simulink model "nonlin_model"  (Simulink 7.3)
settings: Solver=ode113  SolverMode=SingleTasking  StartTime=0  StopTime=0.02  RelTol=1e-3  AbsTol=1e-3
libraries: simulink x3
settings Model: Creator=gladkikh  LastModifiedBy=cubesun  BufferReuse=off
settings SolverCC: ZeroCrossAlgorithm=Adaptive
settings DataIOCC: LimitDataPoints=off  SignalLoggingName=sigsOut
settings OptimizationCC: BlockReduction=off  BooleanDataType=off  InlineParams=on  BufferReuse=off  InitFltsAndDblsToZero=on
settings DebuggingCC: AlgebraicLoopMsg=none  SaveWithParameterizedLinksMsg=none  SignalResolutionControl=TryResolveAllWithWarning  SolverPrmCheckMsg=none  MultiTaskDSMMsg=warning  MultiTaskCondExecSysMsg=none  UnconnectedInputMsg=none  UnconnectedOutputMsg=none  UnconnectedLineMsg=none  StrictBusMsg=None
settings HardwareCC: TargetEndianess=LittleEndian  TargetHWDeviceType=MATLAB Host  ProdEqTarget=off
settings RTWCC: IncludeERTFirstTime=on
settings GRTTargetCC: TargetFcnLib=ansi_tfl_tmw.mat

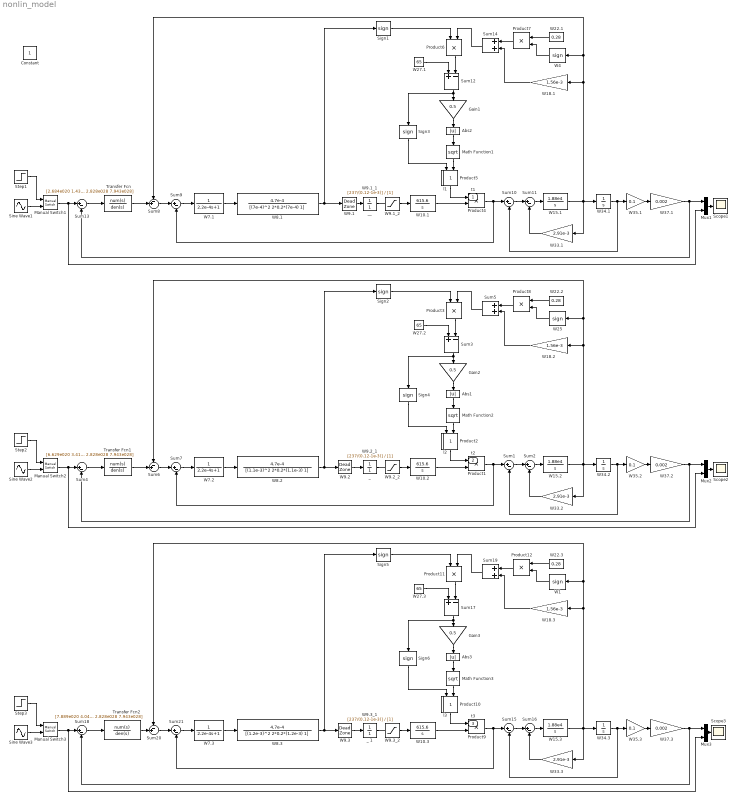
== system nonlin_model ==
  " W9.1_1" : TransferFcn  Numerator=[237/(0.12-1e-3)]  Denominator=[1]
  " W9.2_1" : TransferFcn  Numerator=[237/(0.12-1e-3)]  Denominator=[1]
  " W9.3_1" : TransferFcn  Numerator=[237/(0.12-1e-3)]  Denominator=[1]
  Abs1 : Abs  SaturateOnIntegerOverflow=on
  Abs2 : Abs  SaturateOnIntegerOverflow=on
  Abs3 : Abs  SaturateOnIntegerOverflow=on
  Gain1 : Gain  Gain=0.5  ParameterDataType=sfix(16)  ParameterScaling=2^0  OutDataType=sfix(16)  OutScaling=2^0  SaturateOnIntegerOverflow=on  OutDataTypeStr=Inherit: Same as input  ParamDataTypeStr=Inherit: Same as input
  Gain2 : Gain  Gain=0.5  ParameterDataType=sfix(16)  ParameterScaling=2^0  OutDataType=sfix(16)  OutScaling=2^0  SaturateOnIntegerOverflow=on  OutDataTypeStr=Inherit: Same as input  ParamDataTypeStr=Inherit: Same as input
  Gain3 : Gain  Gain=0.5  ParameterDataType=sfix(16)  ParameterScaling=2^0  OutDataType=sfix(16)  OutScaling=2^0  SaturateOnIntegerOverflow=on  OutDataTypeStr=Inherit: Same as input  ParamDataTypeStr=Inherit: Same as input
  Manual Switch1 : simulink/Signal Routing/Manual Switch  SystemSampleTime=-1  sw=1  action=0  varsize=off
  Manual Switch2 : simulink/Signal Routing/Manual Switch  SystemSampleTime=-1  sw=0  action=0  varsize=off
  Manual Switch3 : simulink/Signal Routing/Manual Switch  SystemSampleTime=-1  sw=0  action=0  varsize=off
  Math Function1 : Math  Operator=sqrt  OutDataType=sfix(16)  OutScaling=2^0  SaturateOnIntegerOverflow=on
  Math Function2 : Math  Operator=sqrt  OutDataType=sfix(16)  OutScaling=2^0  SaturateOnIntegerOverflow=on
  Math Function3 : Math  Operator=sqrt  OutDataType=sfix(16)  OutScaling=2^0  SaturateOnIntegerOverflow=on
  Mux1 : Mux  Inputs=2
  Mux2 : Mux  Inputs=2
  Mux3 : Mux  Inputs=2
  Product{1..12} (12 alike) : Product  OutDataType=sfix(16)  OutScaling=2^0  SaturateOnIntegerOverflow=on  InputSameDT=on  OutDataTypeStr=Inherit: Same as first input
  Scope1 : Scope
      settings: TimeRange=0.01  YMin=0.985  YMax=1.035
  Scope2 : Scope
      settings: YMin=-1  YMax=1
  Scope3 : Scope
      settings: YMin=-1  YMax=1  SaveName=ScopeData2
  Sign{1..6} (6 alike) : Signum
  Sine Wave1 : Sin  Amplitude=1  Bias=0  Frequency=3100  Phase=0  Samples=10  SampleTime=0  Offset=0
  Sine Wave2 : Sin  Amplitude=1  Bias=0  Frequency=3100  Phase=0  Samples=10  SampleTime=0  Offset=0
  Sine Wave3 : Sin  Amplitude=1  Bias=0  Frequency=3100  Phase=0  Samples=10  SampleTime=0  Offset=0
  Step1 : Step  Time=0  SampleTime=0
  Step2 : Step  Time=0  SampleTime=0
  Step3 : Step  Time=0  SampleTime=0
  Sum{1..2,4,7,9..11,13,15..16,18,21} (12 alike) : Sum  Inputs=|+-  OutDataType=fixdt(1, 16)  OutScaling=2^0
  Sum12 : Sum  Inputs=+-  OutDataType=sfix(16)  OutScaling=2^0  SaturateOnIntegerOverflow=on  InputSameDT=on  OutDataTypeStr=Inherit: Same as first input
  Sum14 : Sum  OutDataType=sfix(16)  OutScaling=2^0  SaturateOnIntegerOverflow=on  InputSameDT=on  OutDataTypeStr=Inherit: Same as first input
  Sum17 : Sum  Inputs=+-  OutDataType=sfix(16)  OutScaling=2^0  SaturateOnIntegerOverflow=on  InputSameDT=on  OutDataTypeStr=Inherit: Same as first input
  Sum19 : Sum  OutDataType=sfix(16)  OutScaling=2^0  SaturateOnIntegerOverflow=on  InputSameDT=on  OutDataTypeStr=Inherit: Same as first input
  Sum20 : Sum  Inputs=-+|  OutDataType=fixdt(1, 16)  OutScaling=2^0
  Sum3 : Sum  Inputs=+-  OutDataType=sfix(16)  OutScaling=2^0  SaturateOnIntegerOverflow=on  InputSameDT=on  OutDataTypeStr=Inherit: Same as first input
  Sum5 : Sum  OutDataType=sfix(16)  OutScaling=2^0  SaturateOnIntegerOverflow=on  InputSameDT=on  OutDataTypeStr=Inherit: Same as first input
  Sum6 : Sum  Inputs=-+|  OutDataType=fixdt(1, 16)  OutScaling=2^0
  Sum8 : Sum  Inputs=-+|  OutDataType=fixdt(1, 16)  OutScaling=2^0
  Transfer Fcn : TransferFcn  Numerator=[2.684e020 1.439e024 1.588e027 2.837e030 6.501e032 9.43e034 1.064e037 2.383e036]  Denominator=[1 1.539e006 8.565e011 2.152e017 2.439e022 1.001e027 2.828e028 7.943e028]
  Transfer Fcn1 : TransferFcn  Numerator=[6.629e020 3.416e024 2.457e027 2.993e030 6.686e032 9.562e034 1.64e037 2.383e036]  Denominator=[1 1.539e006 8.565e011 2.152e017 2.439e022 1.001e027 2.828e028 7.943e028]
  Transfer Fcn2 : TransferFcn  Numerator=[7.889e020 4.041e024 2.705e027 3.036e030 6.736e032 9.595e034 1.064e037 2.383e036]  Denominator=[1 1.539e006 8.565e011 2.152e017 2.439e022 1.001e027 2.828e028 7.943e028]
  W1 : Signum
  W10.1 : TransferFcn  Numerator=[615.6]  Denominator=[1 0]
  W10.2 : TransferFcn  Numerator=[615.6]  Denominator=[1 0]
  W10.3 : TransferFcn  Numerator=[615.6]  Denominator=[1 0]
  W15.1 : TransferFcn  Numerator=[1.88e4]  Denominator=[1 0]
  W15.2 : TransferFcn  Numerator=[1.88e4]  Denominator=[1 0]
  W15.3 : TransferFcn  Numerator=[1.88e4]  Denominator=[1 0]
  W18.1 : Gain  Gain=1.56e-3  ParameterDataType=sfix(16)  ParameterScaling=2^0  OutDataType=sfix(16)  OutScaling=2^0  SaturateOnIntegerOverflow=on  OutDataTypeStr=Inherit: Same as input  ParamDataTypeStr=Inherit: Same as input
  W18.2 : Gain  Gain=1.56e-3  ParameterDataType=sfix(16)  ParameterScaling=2^0  OutDataType=sfix(16)  OutScaling=2^0  SaturateOnIntegerOverflow=on  OutDataTypeStr=Inherit: Same as input  ParamDataTypeStr=Inherit: Same as input
  W18.3 : Gain  Gain=1.56e-3  ParameterDataType=sfix(16)  ParameterScaling=2^0  OutDataType=sfix(16)  OutScaling=2^0  SaturateOnIntegerOverflow=on  OutDataTypeStr=Inherit: Same as input  ParamDataTypeStr=Inherit: Same as input
  W22.1 : Constant  Value=0.28  OutDataType=sfix(16)  OutScaling=2^0
  W22.2 : Constant  Value=0.28  OutDataType=sfix(16)  OutScaling=2^0
  W22.3 : Constant  Value=0.28  OutDataType=sfix(16)  OutScaling=2^0
  W25 : Signum
  W27.1 : Constant  Value=65  OutDataType=sfix(16)  OutScaling=2^0
  W27.2 : Constant  Value=65  OutDataType=sfix(16)  OutScaling=2^0
  W27.3 : Constant  Value=65  OutDataType=sfix(16)  OutScaling=2^0
  W33.1 : Gain  Gain=2.91e-3  ParameterDataType=sfix(16)  ParameterScaling=2^0  OutDataType=sfix(16)  OutScaling=2^0  SaturateOnIntegerOverflow=on  OutDataTypeStr=Inherit: Same as input  ParamDataTypeStr=Inherit: Same as input
  W33.2 : Gain  Gain=2.91e-3  ParameterDataType=sfix(16)  ParameterScaling=2^0  OutDataType=sfix(16)  OutScaling=2^0  SaturateOnIntegerOverflow=on  OutDataTypeStr=Inherit: Same as input  ParamDataTypeStr=Inherit: Same as input
  W33.3 : Gain  Gain=2.91e-3  ParameterDataType=sfix(16)  ParameterScaling=2^0  OutDataType=sfix(16)  OutScaling=2^0  SaturateOnIntegerOverflow=on  OutDataTypeStr=Inherit: Same as input  ParamDataTypeStr=Inherit: Same as input
  W34.1 : Integrator
  W34.2 : Integrator
  W34.3 : Integrator
  W35.1 : Gain  Gain=0.1  ParameterDataType=fixdt(1, 16)  ParameterScaling=2^0  OutDataType=fixdt(1, 16)  OutScaling=2^0
  W35.2 : Gain  Gain=0.1  ParameterDataType=fixdt(1, 16)  ParameterScaling=2^0  OutDataType=fixdt(1, 16)  OutScaling=2^0
  W35.3 : Gain  Gain=0.1  ParameterDataType=fixdt(1, 16)  ParameterScaling=2^0  OutDataType=fixdt(1, 16)  OutScaling=2^0
  W37.1 : Gain  Gain=0.002  ParameterDataType=fixdt(1, 16)  ParameterScaling=2^0  OutDataType=fixdt(1, 16)  OutScaling=2^0
  W37.2 : Gain  Gain=0.002  ParameterDataType=fixdt(1, 16)  ParameterScaling=2^0  OutDataType=fixdt(1, 16)  OutScaling=2^0
  W37.3 : Gain  Gain=0.002  ParameterDataType=fixdt(1, 16)  ParameterScaling=2^0  OutDataType=fixdt(1, 16)  OutScaling=2^0
  W4 : Signum
  W7.1 : TransferFcn  Denominator=[2.2e-4 1]
  W7.2 : TransferFcn  Denominator=[2.2e-4 1]
  W7.3 : TransferFcn  Denominator=[2.2e-4 1]
  W8.1 : TransferFcn  Numerator=[4.7e-4]  Denominator=[(7e-4)^2 2*0.2*(7e-4) 1]
  W8.2 : TransferFcn  Numerator=[4.7e-4]  Denominator=[(1.1e-3)^2 2*0.2*(1.1e-3) 1]
  W8.3 : TransferFcn  Numerator=[4.7e-4]  Denominator=[(1.2e-3)^2 2*0.2*(1.2e-3) 1]
  W9.1 : DeadZone  LowerValue=-1e-3  UpperValue=1e-3  SaturateOnIntegerOverflow=on
  W9.1_2 : Saturate  UpperLimit=237  LowerLimit=-237
  W9.2 : DeadZone  LowerValue=-1e-3  UpperValue=1e-3  SaturateOnIntegerOverflow=on
  W9.2_2 : Saturate  UpperLimit=237  LowerLimit=-237
  W9.3 : DeadZone  LowerValue=-1e-3  UpperValue=1e-3  SaturateOnIntegerOverflow=on
  W9.3_2 : Saturate  UpperLimit=237  LowerLimit=-237
  "_ " : TransferFcn  Numerator=1  Denominator=[1]
  _ 1 : TransferFcn  Numerator=1  Denominator=[1]
  "__ " : TransferFcn  Numerator=1  Denominator=[1]
  l1 : Constant  OutDataType=sfix(16)  OutScaling=2^0
  l2 : Constant  OutDataType=sfix(16)  OutScaling=2^0
  l3 : Constant  OutDataType=sfix(16)  OutScaling=2^0
  t1 : Outport  OutDataType=fixdt(1, 16)  OutScaling=2^0
  t2 : Outport  Port=2  OutDataType=fixdt(1, 16)  OutScaling=2^0
  t3 : Outport  Port=3  OutDataType=fixdt(1, 16)  OutScaling=2^0
  Constant : Constant  IOType=siggen  OutDataType=sfix(16)  OutScaling=2^0
  wires:
  Manual Switch1/1 -> Sum13/1, Mux1/2
  Step1/1 -> Manual Switch1/1
  Sum9/1 -> W7.1/1
  W15.1/1 -> W34.1/1, W33.1/1, W18.1/1, Sum8/1, W4/1
  Math Function1/1 -> Product5/2
  W8.1/1 -> Sign1/1, W9.1/1
  Gain1/1 -> Abs2/1
  Abs2/1 -> Math Function1/1
  Sum12/1 -> Gain1/1, Sign3/1
  W22.1/1 -> Product7/1
  W7.1/1 -> W8.1/1
  Product6/1 -> Sum12/2
  W27.1/1 -> Sum12/1
  Sine Wave1/1 -> Manual Switch1/2
  Mux1/1 -> Scope1/1
  W33.1/1 -> Sum11/2
  Sum11/1 -> W15.1/1
  Sum10/1 -> Sum11/1
  Sum8/1 -> Sum9/1
  W34.1/1 -> W35.1/1, Sum10/2
  Sum14/1 -> Product6/2
  Product7/1 -> Sum14/1
  W18.1/1 -> Sum14/2
  Sum13/1 -> Transfer Fcn/1
  Product4/1 -> Sum10/1, Sum9/2
  W10.1/1 -> Product4/2
  Sign1/1 -> Product6/1
  Sign3/1 -> Product5/1
  W4/1 -> Product7/2
  Transfer Fcn/1 -> Sum8/2
  l1/1 -> Product4/1
  Product5/1 -> t1/1
  W35.1/1 -> W37.1/1
  W37.1/1 -> Mux1/1, Sum13/2
  W9.1/1 -> "__ "/1
  "__ "/1 -> W10.1/1
  " W9.1_1"/1 -> " W9.1_1"/1
  W9.1_2/1 -> W9.1_2/1
  Manual Switch2/1 -> Sum4/1, Mux2/2
  Step2/1 -> Manual Switch2/1
  Sum7/1 -> W7.2/1
  W15.2/1 -> W34.2/1, W33.2/1, W18.2/1, Sum6/1, W25/1
  Math Function2/1 -> Product2/2
  W8.2/1 -> Sign2/1, W9.2/1
  Gain2/1 -> Abs1/1
  Abs1/1 -> Math Function2/1
  Sum3/1 -> Gain2/1, Sign4/1
  W22.2/1 -> Product8/1
  W7.2/1 -> W8.2/1
  Product3/1 -> Sum3/2
  W27.2/1 -> Sum3/1
  Sine Wave2/1 -> Manual Switch2/2
  Mux2/1 -> Scope2/1
  W33.2/1 -> Sum2/2
  Sum2/1 -> W15.2/1
  Sum1/1 -> Sum2/1
  Sum6/1 -> Sum7/1
  W34.2/1 -> W35.2/1, Sum1/2
  Sum5/1 -> Product3/2
  Product8/1 -> Sum5/1
  W18.2/1 -> Sum5/2
  Sum4/1 -> Transfer Fcn1/1
  Product1/1 -> Sum1/1, Sum7/2
  W10.2/1 -> Product1/2
  Sign2/1 -> Product3/1
  Sign4/1 -> Product2/1
  W25/1 -> Product8/2
  Transfer Fcn1/1 -> Sum6/2
  l2/1 -> Product1/1
  Product2/1 -> t2/1
  W35.2/1 -> W37.2/1
  W37.2/1 -> Mux2/1, Sum4/2
  W9.2/1 -> "_ "/1
  "_ "/1 -> W10.2/1
  " W9.2_1"/1 -> " W9.2_1"/1
  W9.2_2/1 -> W9.2_2/1
  Manual Switch3/1 -> Sum18/1, Mux3/2
  Step3/1 -> Manual Switch3/1
  Sum21/1 -> W7.3/1
  W15.3/1 -> W34.3/1, W33.3/1, W18.3/1, Sum20/1, W1/1
  Math Function3/1 -> Product10/2
  W8.3/1 -> Sign5/1, W9.3/1
  Gain3/1 -> Abs3/1
  Abs3/1 -> Math Function3/1
  Sum17/1 -> Gain3/1, Sign6/1
  W22.3/1 -> Product12/1
  W7.3/1 -> W8.3/1
  Product11/1 -> Sum17/2
  W27.3/1 -> Sum17/1
  Sine Wave3/1 -> Manual Switch3/2
  Mux3/1 -> Scope3/1
  W33.3/1 -> Sum16/2
  Sum16/1 -> W15.3/1
  Sum15/1 -> Sum16/1
  Sum20/1 -> Sum21/1
  W34.3/1 -> W35.3/1, Sum15/2
  Sum19/1 -> Product11/2
  Product12/1 -> Sum19/1
  W18.3/1 -> Sum19/2
  Sum18/1 -> Transfer Fcn2/1
  Product9/1 -> Sum15/1, Sum21/2
  W10.3/1 -> Product9/2
  Sign5/1 -> Product11/1
  Sign6/1 -> Product10/1
  W1/1 -> Product12/2
  Transfer Fcn2/1 -> Sum20/2
  l3/1 -> Product9/1
  Product10/1 -> t3/1
  W35.3/1 -> W37.3/1
  W37.3/1 -> Mux3/1, Sum18/2
  W9.3/1 -> _ 1/1
  _ 1/1 -> W10.3/1
  " W9.3_1"/1 -> " W9.3_1"/1
  W9.3_2/1 -> W9.3_2/1
